simulink model "fig_5_6"  (R2021b)
settings: Solver=ode23t  StartTime=0.0  StopTime=0.1  FixedStep=1e-5  RelTol=1e-4  EnableMultiTasking=on
undefined symbols (not defined in the file): Ts
libraries: spsSeriesRLCBranchLib x3, spsDiodeLib x1, spsMosfetLib x1, spsMultimeterLib x1, spsDCVoltageSourceLib x1, spspowerguiLib x1
settings Model: Creator=umi  LastModifiedBy=DELL
settings SolverCC: AlgebraicLoopSolver=TrustRegion
settings DataIOCC: LimitDataPoints=on  SaveFormat=Array  ReturnWorkspaceOutputs=off
settings OptimizationCC: LifeSpan=inf
settings DebuggingCC: SolverPrmCheckMsg=warning  SFUnexpectedBacktrackingDiag=warning  SFNoUnconditionalDefaultTransitionDiag=warning  SFExecutionAtInitializationDiag=none  SFMachineParentedDataDiag=warning  ArithmeticOperatorsInVariantConditions=warning
settings HardwareCC: ProdBitPerPointer=32  ProdBitPerSizeT=32  ProdBitPerPtrDiffT=32  ProdLargestAtomicFloat=None  ProdIntDivRoundTo=Undefined  ProdEndianess=Unspecified  ProdWordSize=32  ProdHWDeviceType=32-bit Generic
settings ModelReferenceCC: PropagateSignalLabelsOutOfModel=off
settings SFSimCC: SimUseLocalCustomCode=off  CustomCodeUndefinedFunction=UseInterfaceOnly
settings RTWCC: RTWUseLocalCustomCode=off
settings CodeAppCC: StateflowObjectComments=on
settings GRTTargetCC: TargetLangStandard=C89/C90 (ANSI)
settings ConfigComp: CovMetricSettings=dw  CovSaveCumulativeToWorkspaceVar=on  CovSaveSingleToWorkspaceVar=on  CovExternalEMLEnable=off  CovSFcnEnable=off
settings SimscapeCC: SimscapeNormalizeSystem=off

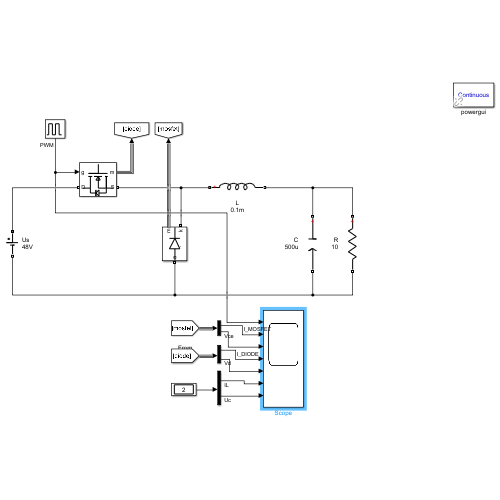
[thumbnail: Simulink's stored preview of the top-level diagram]
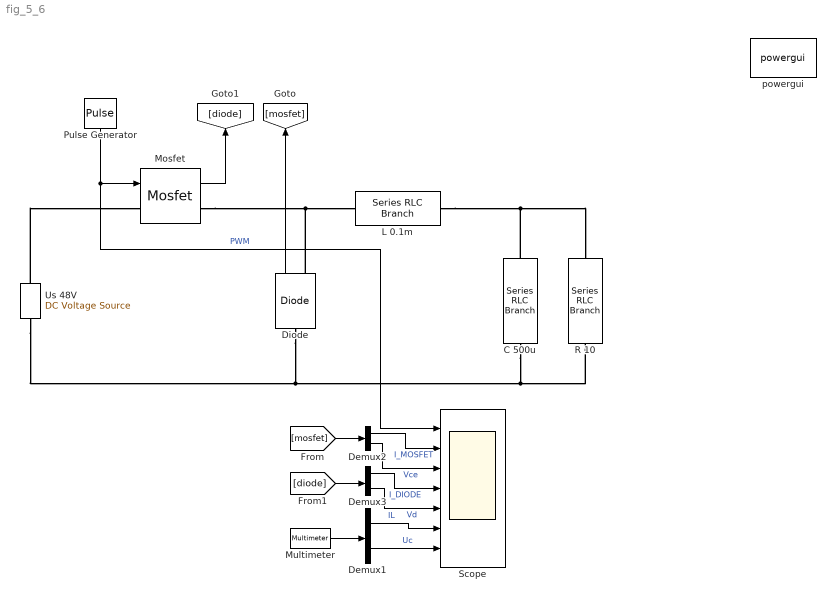
== system fig_5_6 ==
  C 500u : spsSeriesRLCBranchLib/Series RLC Branch  LConnTagsString=__new0  RConnTagsString=__new0  BranchType=C  Resistance=1  Inductance=1e-3  SetiL0=off  InitialCurrent=0  Capacitance=500e-6  Setx0=off  InitialVoltage=0  Measurements=Branch voltage
  Demux1 : Demux  Outputs=2
  Demux2 : Demux  Outputs=2
  Demux3 : Demux  Outputs=2
  Diode : spsDiodeLib/Diode  Ron=0.001  Lon=1e-8  Vf=0.7  IC=0  UseSnubber=off  Rs=1e5  Cs=Inf  Measurements=on
  L 0.1m : spsSeriesRLCBranchLib/Series RLC Branch  LConnTagsString=__new0  RConnTagsString=__new0  BranchType=L  Resistance=1  Inductance=1e-4  SetiL0=off  InitialCurrent=0  Capacitance=1e-6  Setx0=off  InitialVoltage=0  Measurements=Branch voltage and current
  Mosfet : spsMosfetLib/Mosfet  Ron=0.1  Lon=0  Rd=0.01  Vfd=0  IC=0  Rs=1e5  Cs=inf  Measurements=on
  Multimeter : spsMultimeterLib/Multimeter  PhasorSimulation=off  OutputType=Complex  sel=[3 1]  L=4  Gain=[1 1]  yselected={'Ib: L 0.1m','Ub: C 500u'};  PSBOutputType=1  PSBequivalent=0  AxesSetting=[0,0.1,-100,100]  Display=0  SavedBlockNames=-11
  Pulse Generator : DiscretePulseGenerator  PulseType=Time based  Period=25e-6  PulseWidth=25
  R 10 : spsSeriesRLCBranchLib/Series RLC Branch  LConnTagsString=__new0  RConnTagsString=__new0  BranchType=R  Resistance=10  Inductance=1e-3  SetiL0=off  InitialCurrent=0  Capacitance=1e-6  Setx0=off  InitialVoltage=0  Measurements=Branch current
  Scope : Scope  NumInputPorts=7
  Us 48V : spsDCVoltageSourceLib/DC Voltage Source  Amplitude=48  Measurements=None
  powergui : spspowerguiLib/powergui  Priority=1  SimulationMode=Continuous  SampleTime=Ts  frequency=60  Iterations=50  frequencyindice=0  Pbase=100e6  ErrMax=1e-4  UnitsV=kV  UnitsW=MW  buscounter=0  FunctionMessages=off  echomessages=off  EnableUseOfTLC=off  CurrentSourceSwitches=off  DisableSnubberDevices=on  DisableRonSwitches=off  DisableVfSwitches=off  DisplayEquations=off  AutomaticDiscreteSolvers=off  SolverType=Tustin/Backward Euler (TBE)  Interpol=off  ExternalGateDelay=off  methode=off  Ts=100  x0status=blocks  SPID=on  SwTol=0  HookPort=off  NonlinearTolerance=1e-4  nMaxIteration=100  ContinueOnMaxIteration=off  RestoreLinks=warning  ResistiveCurrentMeasurement=off  Frange=[0:2:500]  Ylog=off  Xlog=on  ShowGrid=off  save=off  variable=ZData  structure=0  ZoomFFT=off  StartTime=0.0  cycles=1  DisplayStyle=1  fundamental=60  FreqAxis=off  MaxFrequency=1000  frequencyindicesteady=1  RmsSteady=1  display=off
  wires:
  [mosfet] -> Demux2/1
  Demux2/1 -> Scope/2  "I_MOSFET"
  [diode] -> Demux3/1
  Demux3/1 -> Scope/4  "I_DIODE"
  Multimeter/1 -> Demux1/1
  Diode/1 -> [mosfet]
  Mosfet/1 -> [diode]
  Pulse Generator/1 -> Mosfet/1, Scope/1  "PWM"
  Demux1/1 -> Scope/6  "IL"
  Demux1/2 -> Scope/7  "Uc"
  Demux3/2 -> Scope/5  "Vd"
  Demux2/2 -> Scope/3  "Vce"
  connections:
  Us 48V/RConn1 -- Mosfet/LConn1
  Mosfet/RConn1 -- Diode/RConn1 -- L 0.1m/LConn1
  Us 48V/LConn1 -- Diode/LConn1 -- R 10/RConn1 -- C 500u/RConn1
  L 0.1m/RConn1 -- R 10/LConn1 -- C 500u/LConn1
